simulink model "Quadrotor_PID"  (R2023a)
settings: Solver=VariableStepAuto  StartTime=0.0  StopTime=2000  RelTol=1e-3
model workspace (MAT data in the model file):
  b = 0.000142
  g = 9.8
  m = 1
undefined symbols (not defined in the file or in its folder): Earth, Pitch, Receive, Roll, Send, WGS84, X, Y, Yaw, Z
libraries: slpidlib x6, aerolibfltsims x3, aerolibtransform2 x1
settings Model: Creator=huawei  LastModifiedBy=User
settings SolverCC: ZeroCrossAlgorithm=Adaptive  AlgebraicLoopSolver=TrustRegion
settings DebuggingCC: IgnoredZcDiagnostic=none  UnconnectedInputMsg=warning  UnconnectedOutputMsg=warning  UnconnectedLineMsg=warning
settings ModelReferenceCC: EnableRefExpFcnMdlSchedulingChecks=on
settings RTWCC: DLArmComputeVersion=19.05

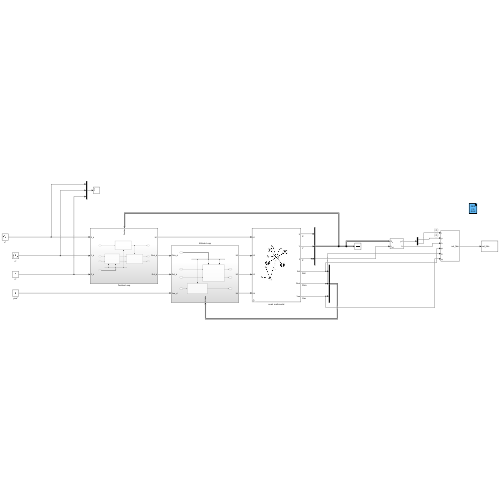
[thumbnail: Simulink's stored preview of the top-level diagram]
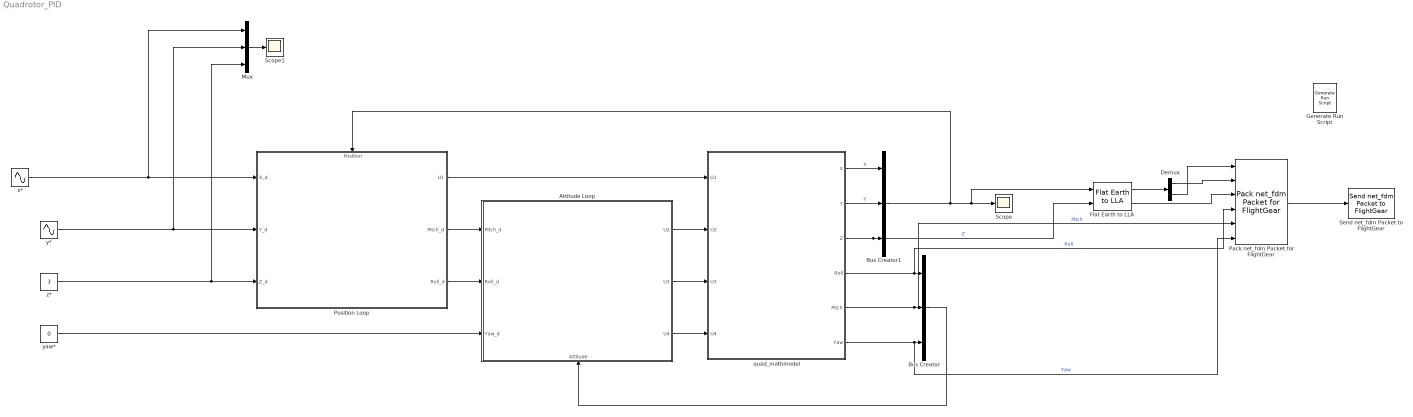
== system Quadrotor_PID ==
  Attitude Loop : Subsystem
      settings: PortSchema="{\"entries\":[{\"content\":{\"sides\":[{\"content\":{\"connectorIds\":[\"In1\",\"In2\",\"In3\"]},\"type\":\"ConnectorPlacement.EquallySpacedRectSide\",\"uuid\":\"741c63cb-3193-49ed-b6fe-0554dd8eb38b\"},{\"content\":{\"connectorIds\":[\"Out1\",\"Out2\",\"Out3\"],\"side\":\"RIGHT\"},\"type\":\"ConnectorPlacement.EquallySpacedRectSide\",\"uuid\":\"55d4e1d6-ced0-4d00-88f3-94ecae3eab08\"},{\"content\":{\"connectorIds\":[],\"side\":\"TOP\"},\"type\":\"ConnectorPlacement.EquallySpacedRectSide\",\"uuid\":\"670d5dfa-1a50-4aee-963c-097076b25aa9\"},{\"content\":{\"connectorIds\":[\"In4\"],\"side\":\"BOTTOM\"},\"type\":\"ConnectorPlacement.EquallySpacedRectSide\",\"uuid\":\"461487f9-9010-46f7-8d40-b6bfcadca1df\"},{\"content\":{\"connectorIds\":[],\"side\":\"HIDDEN\"},\"type\":\"ConnectorPlacement.EquallySpacedRectSide\",\"uuid\":\"46070c40-0b01-41e4-9178-eaa0a7804a93\"}]},\"type\":\"ConnectorPlacement.EquallySpacedConnector\",\"uuid\":\"b0fd4550-2f46-4562-9b6e-a30bcd34312f\"}],\"packageUris\":[\"http://schema.mathworks.com/mf0/Connector/R2020b\"],\"version\":\"1.0\"}"
  Bus Creator : BusCreator  Inputs=Roll,Pitch,Yaw
  Bus Creator1 : BusCreator  Inputs=X,Y,Z
  Demux : Demux  Outputs=2
  Flat Earth to LLA : aerolibtransform2/Flat Earth to LLA  units=Metric (MKS)  ptype=Earth (WGS84)  F=1/298.257223563  R=6378137  refPosPort=off  LL0=[0 10]  psi=0
  Generate Run Script : aerolibfltsims/Generate Run Script  Architecture=Default  dataFlow=Send-Receive  GeometryModelName=c172p  AirportId=KSFO  RunwayId=10L  InitialAltitude=0  InitialHeading=113  OffsetDistance=0  OffsetAzimuth=0  InstallScenery=off  DisableShaders=off  OriginAddress=127.0.0.1  DestinationPort=5502  OriginPort=5505  LocalAddress=127.0.0.1  OutputFileName=runfg.bat  FlightGearBaseDirectory=C:\Program Files\FlightGear 2020.3
  Mux : Mux  Inputs=3
  Pack net_fdm Packet for FlightGear : aerolibfltsims/Pack net_fdm Packet for FlightGear  FlightGearVersion=v2019.1  ShowPositionAttitudeInputs=on  ShowVelocityAccelerationInputs=off  ShowControlSurfacePositionInputs=off  ShowEngineFuelInputs=off  ShowLandingGearInputs=off  ShowEnvironmentInputs=off  SampleTime=-1  packetVersion=24
  Position Loop : Subsystem
      settings: PortSchema="{\"entries\":[{\"content\":{\"sides\":[{\"content\":{\"connectorIds\":[\"In1\",\"In2\",\"In3\"]},\"type\":\"ConnectorPlacement.EquallySpacedRectSide\",\"uuid\":\"741c63cb-3193-49ed-b6fe-0554dd8eb38b\"},{\"content\":{\"connectorIds\":[\"Out1\",\"Out2\",\"Out3\"],\"side\":\"RIGHT\"},\"type\":\"ConnectorPlacement.EquallySpacedRectSide\",\"uuid\":\"55d4e1d6-ced0-4d00-88f3-94ecae3eab08\"},{\"content\":{\"connectorIds\":[\"In4\"],\"side\":\"TOP\"},\"type\":\"ConnectorPlacement.EquallySpacedRectSide\",\"uuid\":\"670d5dfa-1a50-4aee-963c-097076b25aa9\"},{\"content\":{\"connectorIds\":[],\"side\":\"BOTTOM\"},\"type\":\"ConnectorPlacement.EquallySpacedRectSide\",\"uuid\":\"31dc6e32-e4ae-4a63-8318-e80959689dd0\"},{\"content\":{\"connectorIds\":[],\"side\":\"HIDDEN\"},\"type\":\"ConnectorPlacement.EquallySpacedRectSide\",\"uuid\":\"46070c40-0b01-41e4-9178-eaa0a7804a93\"}]},\"type\":\"ConnectorPlacement.EquallySpacedConnector\",\"uuid\":\"b0fd4550-2f46-4562-9b6e-a30bcd34312f\"}],\"packageUris\":[\"http://schema.mathworks.com/mf0/Connector/R2020b\"],\"version\":\"1.0\"}"
  Scope : Scope
  Scope1 : Scope
  Send net_fdm Packet to FlightGear : aerolibfltsims/Send net_fdm Packet to FlightGear  DestinationIpAddress=127.0.0.1  DestinationPort=5502  LocalIpPort=-1  varLen=off  SampleTime=-1
  quad_mathmodel : Subsystem  mask{m=1, L=0.24, b=1.42e-4, d=6.21e-5, g=9.8, Ix=8.1e-3, Iy=8.1e-3, Iz=12.4e-3, Jtp=7.24e-5}
      mask DialogControl ParameterGroupVar Prompt: 四旋翼飞行器参数设置
      mask DialogControl Container10 Prompt: 飞行器质量(kg)
      mask DialogControl Container11 Prompt: 质心到电机中心轴距(m)
      mask DialogControl Container16 Prompt: 升力系数
      mask DialogControl Container15 Prompt: 阻力系数
      mask DialogControl Container14 Prompt: 重力加速度
      mask DialogControl Container13 Prompt: 绕X轴转动惯量
      mask DialogControl Container12 Prompt: 绕Y轴转动惯量
      mask DialogControl Container17 Prompt: 绕Z轴转动惯量
      mask DialogControl Container18 Prompt: 机体绕转轴的总转动惯量（可忽略）
      mask Display: image('$imagefile'); % Use "Edit Image" on toolstrip to change.
  x* : Sin  Frequency=2*pi*.003  Phase=-pi/2  SampleTime=0
  y* : Sin  Frequency=2*pi*.003  SampleTime=0
  yaw* : Constant  Value=0
  z* : Constant  Value=3
  wires:
  quad_mathmodel/3(Z) -> Flat Earth to LLA/2, Bus Creator1/3  "Z"
  Bus Creator1/1 -> Flat Earth to LLA/1, Scope/1, Position Loop/4(Position)
  x*/1 -> Mux/1, Position Loop/1(X_d)
  quad_mathmodel/2(Y) -> Bus Creator1/2  "Y"
  Attitude Loop/3(U4) -> quad_mathmodel/4(U4)
  z*/1 -> Mux/3, Position Loop/3(Z_d)
  Attitude Loop/1(U2) -> quad_mathmodel/2(U2)
  y*/1 -> Mux/2, Position Loop/2(Y_d)
  Position Loop/1(U1) -> quad_mathmodel/1(U1)
  Bus Creator/1 -> Attitude Loop/4(Attitude)
  quad_mathmodel/4(Roll) -> Pack net_fdm Packet for FlightGear/4, Bus Creator/1  "Roll"
  Attitude Loop/2(U3) -> quad_mathmodel/3(U3)
  Position Loop/2(Pitch_d) -> Attitude Loop/1(Pitch_d)
  quad_mathmodel/1(X) -> Bus Creator1/1  "X"
  Position Loop/3(Roll_d) -> Attitude Loop/2(Roll_d)
  quad_mathmodel/5(Pitch) -> Pack net_fdm Packet for FlightGear/5, Bus Creator/2  "Pitch"
  yaw*/1 -> Attitude Loop/3(Yaw_d)
  quad_mathmodel/6(Yaw) -> Pack net_fdm Packet for FlightGear/6, Bus Creator/3  "Yaw"
  Mux/1 -> Scope1/1
  Pack net_fdm Packet for FlightGear/1 -> Send net_fdm Packet to FlightGear/1
  Flat Earth to LLA/1 -> Demux/1
  Demux/1 -> Pack net_fdm Packet for FlightGear/2
  Demux/2 -> Pack net_fdm Packet for FlightGear/1
  Flat Earth to LLA/2 -> Pack net_fdm Packet for FlightGear/3

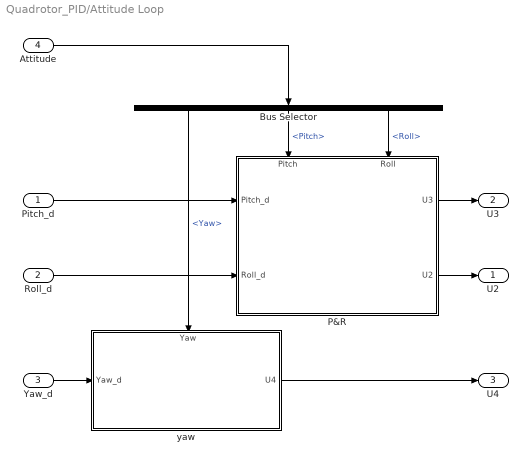
== system Quadrotor_PID/Attitude Loop ==
  Pitch_d : Inport
  Roll_d : Inport  Port=2
  Yaw_d : Inport  Port=3
  Attitude : Inport  Port=4
  Bus Selector : BusSelector  OutputSignals=Yaw,Pitch,Roll
  P&R : Subsystem
      settings: PortSchema="{\"entries\":[{\"content\":{\"sides\":[{\"content\":{\"connectorIds\":[\"In1\",\"In2\"]},\"type\":\"ConnectorPlacement.EquallySpacedRectSide\",\"uuid\":\"5a168f57-9082-4ef9-b723-ec42d235f15b\"},{\"content\":{\"connectorIds\":[\"Out1\",\"Out2\"],\"side\":\"RIGHT\"},\"type\":\"ConnectorPlacement.EquallySpacedRectSide\",\"uuid\":\"1b4dc671-5a32-4537-87d8-64b7817d412d\"},{\"content\":{\"connectorIds\":[\"In3\",\"In4\"],\"side\":\"TOP\"},\"type\":\"ConnectorPlacement.EquallySpacedRectSide\",\"uuid\":\"3d489923-4a97-462b-9fd9-288b2bf2a159\"},{\"content\":{\"connectorIds\":[],\"side\":\"HIDDEN\"},\"type\":\"ConnectorPlacement.EquallySpacedRectSide\",\"uuid\":\"f2e8a974-f6bc-4a20-b9fe-32904cbbc482\"}]},\"type\":\"ConnectorPlacement.EquallySpacedConnector\",\"uuid\":\"91228c47-fce9-4c1d-8a3a-204dc80f90dd\"}],\"packageUris\":[\"http://schema.mathworks.com/mf0/Connector/R2020b\"],\"version\":\"1.0\"}"
  yaw : Subsystem
      settings: PortSchema="{\"entries\":[{\"content\":{\"sides\":[{\"content\":{\"connectorIds\":[\"In1\"]},\"type\":\"ConnectorPlacement.EquallySpacedRectSide\",\"uuid\":\"a7b1533a-1266-40d5-b52c-012082b26468\"},{\"content\":{\"connectorIds\":[\"Out1\"],\"side\":\"RIGHT\"},\"type\":\"ConnectorPlacement.EquallySpacedRectSide\",\"uuid\":\"b4620233-0e85-40ae-9738-c29ba1209ef5\"},{\"content\":{\"connectorIds\":[\"In2\"],\"side\":\"TOP\"},\"type\":\"ConnectorPlacement.EquallySpacedRectSide\",\"uuid\":\"ab9c222c-25de-47f6-b54f-342fd8d0321b\"},{\"content\":{\"connectorIds\":[],\"side\":\"BOTTOM\"},\"type\":\"ConnectorPlacement.EquallySpacedRectSide\",\"uuid\":\"5eacbb93-3d5d-4d57-aaef-fda87c8b1f96\"},{\"content\":{\"connectorIds\":[],\"side\":\"HIDDEN\"},\"type\":\"ConnectorPlacement.EquallySpacedRectSide\",\"uuid\":\"6ed2670f-d779-4b00-b067-d8065a88322b\"}]},\"type\":\"ConnectorPlacement.EquallySpacedConnector\",\"uuid\":\"8cc1c8e9-c992-4e05-8575-ab9d3ec9e6a4\"}],\"packageUris\":[\"http://schema.mathworks.com/mf0/Connector/R2020b\"],\"version\":\"1.0\"}"
  U2 : Outport
  U3 : Outport  Port=2
  U4 : Outport  Port=3
  wires:
  Bus Selector/2 -> P&R/3(Pitch)  "<Pitch>"
  Roll_d/1 -> P&R/2(Roll_d)
  yaw/1(U4) -> U4/1
  Attitude/1 -> Bus Selector/1
  Bus Selector/3 -> P&R/4(Roll)  "<Roll>"
  Pitch_d/1 -> P&R/1(Pitch_d)
  Bus Selector/1 -> yaw/2(Yaw)  "<Yaw>"
  P&R/2(U2) -> U2/1
  P&R/1(U3) -> U3/1
  Yaw_d/1 -> yaw/1(Yaw_d)

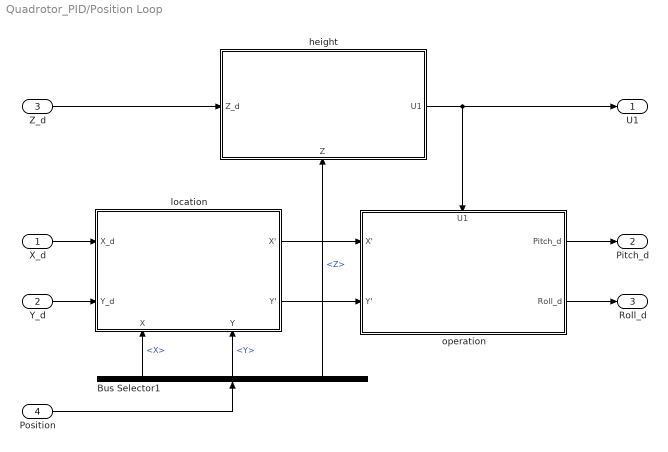
== system Quadrotor_PID/Position Loop ==
  X_d : Inport
  Y_d : Inport  Port=2
  Z_d : Inport  Port=3
  Position : Inport  Port=4
  Bus Selector1 : BusSelector  OutputSignals=X,Y,Z
  height : Subsystem
      settings: PortSchema="{\"entries\":[{\"content\":{\"sides\":[{\"content\":{\"connectorIds\":[\"In1\"]},\"type\":\"ConnectorPlacement.EquallySpacedRectSide\",\"uuid\":\"a7b1533a-1266-40d5-b52c-012082b26468\"},{\"content\":{\"connectorIds\":[\"Out1\"],\"side\":\"RIGHT\"},\"type\":\"ConnectorPlacement.EquallySpacedRectSide\",\"uuid\":\"b4620233-0e85-40ae-9738-c29ba1209ef5\"},{\"content\":{\"connectorIds\":[],\"side\":\"TOP\"},\"type\":\"ConnectorPlacement.EquallySpacedRectSide\",\"uuid\":\"ab9c222c-25de-47f6-b54f-342fd8d0321b\"},{\"content\":{\"connectorIds\":[\"In2\"],\"side\":\"BOTTOM\"},\"type\":\"ConnectorPlacement.EquallySpacedRectSide\",\"uuid\":\"c0ec5864-a2e3-4dc9-86df-2e8e31dc698f\"},{\"content\":{\"connectorIds\":[],\"side\":\"HIDDEN\"},\"type\":\"ConnectorPlacement.EquallySpacedRectSide\",\"uuid\":\"6ed2670f-d779-4b00-b067-d8065a88322b\"}]},\"type\":\"ConnectorPlacement.EquallySpacedConnector\",\"uuid\":\"8cc1c8e9-c992-4e05-8575-ab9d3ec9e6a4\"}],\"packageUris\":[\"http://schema.mathworks.com/mf0/Connector/R2020b\"],\"version\":\"1.0\"}"
  "location " : Subsystem
      settings: PortSchema="{\"entries\":[{\"content\":{\"sides\":[{\"content\":{\"connectorIds\":[\"In1\",\"In2\"]},\"type\":\"ConnectorPlacement.EquallySpacedRectSide\",\"uuid\":\"5a168f57-9082-4ef9-b723-ec42d235f15b\"},{\"content\":{\"connectorIds\":[\"Out1\",\"Out2\"],\"side\":\"RIGHT\"},\"type\":\"ConnectorPlacement.EquallySpacedRectSide\",\"uuid\":\"1b4dc671-5a32-4537-87d8-64b7817d412d\"},{\"content\":{\"connectorIds\":[],\"side\":\"TOP\"},\"type\":\"ConnectorPlacement.EquallySpacedRectSide\",\"uuid\":\"3d489923-4a97-462b-9fd9-288b2bf2a159\"},{\"content\":{\"connectorIds\":[\"In3\",\"In4\"],\"side\":\"BOTTOM\"},\"type\":\"ConnectorPlacement.EquallySpacedRectSide\",\"uuid\":\"ca455ebd-18aa-4cdd-b9a1-332337147b86\"},{\"content\":{\"connectorIds\":[],\"side\":\"HIDDEN\"},\"type\":\"ConnectorPlacement.EquallySpacedRectSide\",\"uuid\":\"f2e8a974-f6bc-4a20-b9fe-32904cbbc482\"}]},\"type\":\"ConnectorPlacement.EquallySpacedConnector\",\"uuid\":\"91228c47-fce9-4c1d-8a3a-204dc80f90dd\"}],\"packageUris\":[\"http://schema.mathworks.com/mf0/Connector/R2020b\"],\"version\":\"1.0\"}"
  operation : Subsystem
      settings: PortSchema="{\"entries\":[{\"content\":{\"sides\":[{\"content\":{\"connectorIds\":[\"In1\",\"In2\"]},\"type\":\"ConnectorPlacement.EquallySpacedRectSide\",\"uuid\":\"7b5ff4eb-d8d0-4c09-9af3-42040e275879\"},{\"content\":{\"connectorIds\":[\"Out1\",\"Out2\"],\"side\":\"RIGHT\"},\"type\":\"ConnectorPlacement.EquallySpacedRectSide\",\"uuid\":\"8346582f-6666-4076-82d0-a237d0151848\"},{\"content\":{\"connectorIds\":[\"In3\"],\"side\":\"TOP\"},\"type\":\"ConnectorPlacement.EquallySpacedRectSide\",\"uuid\":\"392c211c-fa44-4e3a-adf5-1ced3bd87e05\"},{\"content\":{\"connectorIds\":[],\"side\":\"HIDDEN\"},\"type\":\"ConnectorPlacement.EquallySpacedRectSide\",\"uuid\":\"198276da-d589-40b0-b73f-71cfec7294bf\"}]},\"type\":\"ConnectorPlacement.EquallySpacedConnector\",\"uuid\":\"5d751e66-253e-464d-b7a7-9553a5bc15c8\"}],\"packageUris\":[\"http://schema.mathworks.com/mf0/Connector/R2020b\"],\"version\":\"1.0\"}"
  U1 : Outport
  Pitch_d : Outport  Port=2
  Roll_d : Outport  Port=3
  wires:
  "location "/1(X') -> operation/1(X')
  Bus Selector1/3 -> height/2(Z)  "<Z>"
  height/1(U1) -> U1/1, operation/3(U1)
  Bus Selector1/2 -> "location "/4(Y)  "<Y>"
  Z_d/1 -> height/1(Z_d)
  Bus Selector1/1 -> "location "/3(X)  "<X>"
  Position/1 -> Bus Selector1/1
  "location "/2(Y') -> operation/2(Y')
  operation/2(Roll_d) -> Roll_d/1
  X_d/1 -> "location "/1(X_d)
  Y_d/1 -> "location "/2(Y_d)
  operation/1(Pitch_d) -> Pitch_d/1

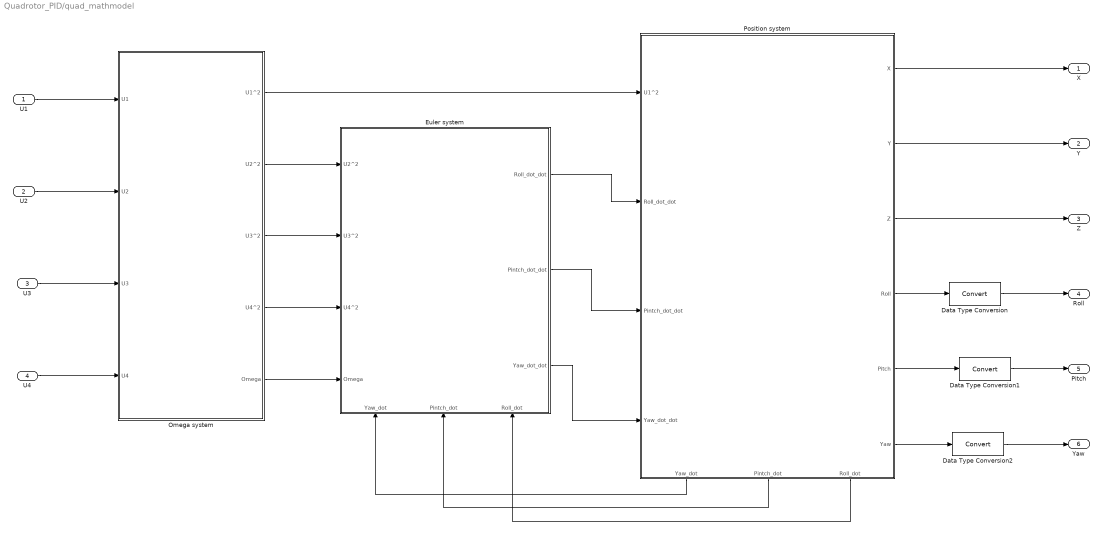
== system Quadrotor_PID/quad_mathmodel ==
  U1 : Inport
  U2 : Inport  Port=2
  U3 : Inport  Port=3
  U4 : Inport  Port=4
  Data Type Conversion : DataTypeConversion  SaturateOnIntegerOverflow=off  RndMeth=Floor
  Data Type Conversion1 : DataTypeConversion  SaturateOnIntegerOverflow=off  RndMeth=Floor
  Data Type Conversion2 : DataTypeConversion  SaturateOnIntegerOverflow=off  RndMeth=Floor
  Euler system : Subsystem
      settings: PortSchema="{\"entries\":[{\"content\":{\"sides\":[{\"content\":{\"connectorIds\":[\"In1\",\"In2\",\"In3\",\"In4\"]},\"type\":\"ConnectorPlacement.EquallySpacedRectSide\",\"uuid\":\"24e9f502-01e2-4796-81d1-4356e5613cd4\"},{\"content\":{\"connectorIds\":[\"Out1\",\"Out2\",\"Out3\"],\"side\":\"RIGHT\"},\"type\":\"ConnectorPlacement.EquallySpacedRectSide\",\"uuid\":\"86fc2a55-a1b7-4625-a7fd-97b1845c6b1e\"},{\"content\":{\"connectorIds\":[],\"side\":\"TOP\"},\"type\":\"ConnectorPlacement.EquallySpacedRectSide\",\"uuid\":\"58e97d03-eced-4c7d-922b-6a4463cc6835\"},{\"content\":{\"connectorIds\":[\"In5\",\"In6\",\"In7\"],\"side\":\"BOTTOM\"},\"type\":\"ConnectorPlacement.EquallySpacedRectSide\",\"uuid\":\"f911275b-2fff-4eb0-817b-81b694121986\"},{\"content\":{\"connectorIds\":[],\"side\":\"HIDDEN\"},\"type\":\"ConnectorPlacement.EquallySpacedRectSide\",\"uuid\":\"f88c6b9c-ef4f-48b0-a4e4-7981c366d7bb\"}]},\"type\":\"ConnectorPlacement.EquallySpacedConnector\",\"uuid\":\"11616862-190a-491d-8e6d-3b18839a1b83\"}],\"packageUris\":[\"http://schema.mathworks.com/mf0/Connector/R2020b\"],\"version\":\"1.0\"}"
  Omega system : Subsystem
  Position system : Subsystem
      settings: PortSchema="{\"entries\":[{\"content\":{\"sides\":[{\"content\":{\"connectorIds\":[\"In1\",\"In2\",\"In3\",\"In4\"]},\"type\":\"ConnectorPlacement.EquallySpacedRectSide\",\"uuid\":\"4e608076-d82c-49dd-b9c3-40de08b530f0\"},{\"content\":{\"connectorIds\":[\"Out1\",\"Out2\",\"Out3\",\"Out4\",\"Out5\",\"Out6\"],\"side\":\"RIGHT\"},\"type\":\"ConnectorPlacement.EquallySpacedRectSide\",\"uuid\":\"79b98a7d-b351-461d-bf57-6a86461ab0e9\"},{\"content\":{\"connectorIds\":[],\"side\":\"TOP\"},\"type\":\"ConnectorPlacement.EquallySpacedRectSide\",\"uuid\":\"a0272396-a878-4308-9d2f-e99a972ffebc\"},{\"content\":{\"connectorIds\":[\"Out7\",\"Out8\",\"Out9\"],\"side\":\"BOTTOM\"},\"type\":\"ConnectorPlacement.EquallySpacedRectSide\",\"uuid\":\"679361ac-afba-4ea2-980e-22b3bd722f7e\"},{\"content\":{\"connectorIds\":[],\"side\":\"HIDDEN\"},\"type\":\"ConnectorPlacement.EquallySpacedRectSide\",\"uuid\":\"68508d46-0468-4fb8-981a-0d305e2aec68\"}]},\"type\":\"ConnectorPlacement.EquallySpacedConnector\",\"uuid\":\"cd6e232c-b153-4628-a51e-54595ea92055\"}],\"packageUris\":[\"http://schema.mathworks.com/mf0/Connector/R2020b\"],\"version\":\"1.0\"}"
  X : Outport
  Y : Outport  Port=2
  Z : Outport  Port=3
  Roll : Outport  Port=4
  Pitch : Outport  Port=5
  Yaw : Outport  Port=6
  wires:
  Position system/6(Yaw) -> Data Type Conversion2/1
  Omega system/5(Omega) -> Euler system/4(Omega)
  Omega system/2(U2^2) -> Euler system/1(U2^2)
  Omega system/3(U3^2) -> Euler system/2(U3^2)
  Position system/2(Y) -> Y/1
  Omega system/1(U1^2) -> Position system/1(U1^2)
  Euler system/2(Pintch_dot_dot) -> Position system/3(Pintch_dot_dot)
  Omega system/4(U4^2) -> Euler system/3(U4^2)
  U3/1 -> Omega system/3(U3)
  Euler system/1(Roll_dot_dot) -> Position system/2(Roll_dot_dot)
  Euler system/3(Yaw_dot_dot) -> Position system/4(Yaw_dot_dot)
  Position system/3(Z) -> Z/1
  U1/1 -> Omega system/1(U1)
  Position system/4(Roll) -> Data Type Conversion/1
  Position system/5(Pitch) -> Data Type Conversion1/1
  Position system/1(X) -> X/1
  U2/1 -> Omega system/2(U2)
  U4/1 -> Omega system/4(U4)
  Position system/9(Roll_dot) -> Euler system/7(Roll_dot)
  Position system/8(Pintch_dot) -> Euler system/6(Pintch_dot)
  Position system/7(Yaw_dot) -> Euler system/5(Yaw_dot)
  Data Type Conversion/1 -> Roll/1
  Data Type Conversion1/1 -> Pitch/1
  Data Type Conversion2/1 -> Yaw/1

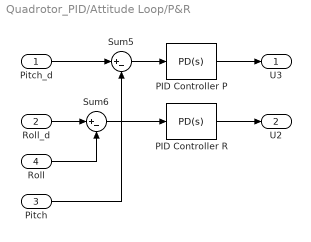
== system Quadrotor_PID/Attitude Loop/P&R ==
  Pitch_d : Inport
  Roll_d : Inport  Port=2
  Pitch : Inport  Port=3
  Roll : Inport  Port=4
  PID Controller P : slpidlib/PID Controller  Controller=PD  Form=Parallel  TimeDomain=Continuous-time  UseExternalTs=off  SampleTime=-1  IntegratorMethod=Forward Euler  FilterMethod=Forward Euler  ControllerParametersSource=internal  P=0.002  I=1.51679966097293e-05  UseKiTs=off  D=0.004  N=3.58143563707461  UseFilter=on  TunerSelectOption=Transfer Function Based (PID Tuner App)  InitialConditionSource=internal  InitialConditionForIntegrator=0  InitialConditionForFilter=0  DifferentiatorICPrevScaledInput=0  ExternalReset=none  TrackingMode=off  Kt=1  LimitOutput=off  SatLimitsSource=internal  UpperSaturationLimit=inf  LowerSaturationLimit=-inf  LinearizeAsGain=on  AntiWindupMode=none  Kb=1  LimitIntegrator=off  UpperIntegratorSaturationLimit=inf  LowerIntegratorSaturationLimit=-inf  POutMin=[]  POutMax=[]  IOutMin=[]  IOutMax=[]  DOutMin=[]  DOutMax=[]  NOutMin=[]  NOutMax=[]  SumOutMin=[]  SumOutMax=[]  SaturationOutMin=[]  SaturationOutMax=[]  PParamMin=[]  PParamMax=[]  IParamMin=[]  IParamMax=[]  DParamMin=[]  DParamMax=[]  NParamMin=[]  NParamMax=[]  KbParamMin=[]  KbParamMax=[]  KtParamMin=[]  KtParamMax=[]  KbOutMin=[]  KbOutMax=[]  KtOutMin=[]  KtOutMax=[]  IntegratorOutMin=[]  IntegratorOutMax=[]  FilterOutMin=[]  FilterOutMax=[]  SumI1OutMin=[]  SumI1OutMax=[]  SumI2OutMin=[]  SumI2OutMax=[]  SumI3OutMin=[]  SumI3OutMax=[]  SumI4OutMin=[]  SumI4OutMax=[]  SumDOutMin=[]  SumDOutMax=[]  DifferentiatorOutMin=[]  DifferentiatorOutMax=[]  FilterDiffOutCoefMin=[]  FilterDiffOutCoefMax=[]  ReciprocalOutMin=[]  ReciprocalOutMax=[]  SumDenOutMin=[]  SumDenOutMax=[]  SumNumOutMin=[]  SumNumOutMax=[]  DivideOutMin=[]  DivideOutMax=[]  UdiffTsProdOutMin=[]  UdiffTsProdOutMax=[]  NTsProdOutMin=[]  NTsProdOutMax=[]  UintegralTsProdOutMin=[]  UintegralTsProdOutMax=[]  UngainTsProdOutMin=[]  UngainTsProdOutMax=[]  ClampingZeroOutDataTypeStr=Inherit: Inherit via back propagation  ClampingZeroOutMin=[]  ClampingZeroOutMax=[]  FilterDenConstantOutDataTypeStr=Inherit: Inherit via back propagation  FilterDenConstantOutMin=[]  FilterDenConstantOutMax=[]  PCopyOutDataTypeStr=Inherit: Inherit via back propagation  PCopyOutMin=[]  PCopyOutMax=[]  NCopyOutDataTypeStr=Inherit: Inherit via back propagation  NCopyOutMin=[]  NCopyOutMax=[]  IntegratorContinuousStateAttributes=''  IntegratorStateMustResolveToSignalObject=off  IntegratorRTWStateStorageClass=Auto  FilterContinuousStateAttributes=''  FilterStateMustResolveToSignalObject=off  FilterRTWStateStorageClass=Auto  ParallelPVariant=InternalParameters  IdealPVariant=Disabled  IVariant=Disabled  DVariant=InternalParameters  IntegratorVariant=Disabled  SatVariant=Disabled  AWVariant=Disabled  PCopyVariant=Disabled  TRVariant=Disabled  FdbkBlocksVariant=Forward  IdealPFdbkVariant=Disabled  SatFdbkVariant=Disabled  DerivativeFilterVariant=ContFilter  NVariant=InternalParameters  NCopyVariant=Disabled  FilterICVariant=InternalICsFilter  IntegratorICVariant=Disabled  ExternalResetVariant=Disabled  TRSumVariant=Passthrough  SumFdbkVariant=Disabled  SumVariant=Sum_PD  TsampFilterVariant=InternalTs  TsampNgainVariant=Passthrough  TsampIntegralVariant=Disabled_SignalSpec  ExternalSaturationOutDataTypeStr=Inherit: Same as second input
  PID Controller R : slpidlib/PID Controller  Controller=PD  Form=Parallel  TimeDomain=Continuous-time  UseExternalTs=off  SampleTime=-1  IntegratorMethod=Forward Euler  FilterMethod=Forward Euler  ControllerParametersSource=internal  P=0.000517944009365722  I=2.09015293720685e-05  UseKiTs=off  D=0.0031516571893313  N=4.69883432592557  UseFilter=on  TunerSelectOption=Transfer Function Based (PID Tuner App)  InitialConditionSource=internal  InitialConditionForIntegrator=0  InitialConditionForFilter=0  DifferentiatorICPrevScaledInput=0  ExternalReset=none  TrackingMode=off  Kt=1  LimitOutput=off  SatLimitsSource=internal  UpperSaturationLimit=inf  LowerSaturationLimit=-inf  LinearizeAsGain=on  AntiWindupMode=none  Kb=1  LimitIntegrator=off  UpperIntegratorSaturationLimit=inf  LowerIntegratorSaturationLimit=-inf  POutMin=[]  POutMax=[]  IOutMin=[]  IOutMax=[]  DOutMin=[]  DOutMax=[]  NOutMin=[]  NOutMax=[]  SumOutMin=[]  SumOutMax=[]  SaturationOutMin=[]  SaturationOutMax=[]  PParamMin=[]  PParamMax=[]  IParamMin=[]  IParamMax=[]  DParamMin=[]  DParamMax=[]  NParamMin=[]  NParamMax=[]  KbParamMin=[]  KbParamMax=[]  KtParamMin=[]  KtParamMax=[]  KbOutMin=[]  KbOutMax=[]  KtOutMin=[]  KtOutMax=[]  IntegratorOutMin=[]  IntegratorOutMax=[]  FilterOutMin=[]  FilterOutMax=[]  SumI1OutMin=[]  SumI1OutMax=[]  SumI2OutMin=[]  SumI2OutMax=[]  SumI3OutMin=[]  SumI3OutMax=[]  SumI4OutMin=[]  SumI4OutMax=[]  SumDOutMin=[]  SumDOutMax=[]  DifferentiatorOutMin=[]  DifferentiatorOutMax=[]  FilterDiffOutCoefMin=[]  FilterDiffOutCoefMax=[]  ReciprocalOutMin=[]  ReciprocalOutMax=[]  SumDenOutMin=[]  SumDenOutMax=[]  SumNumOutMin=[]  SumNumOutMax=[]  DivideOutMin=[]  DivideOutMax=[]  UdiffTsProdOutMin=[]  UdiffTsProdOutMax=[]  NTsProdOutMin=[]  NTsProdOutMax=[]  UintegralTsProdOutMin=[]  UintegralTsProdOutMax=[]  UngainTsProdOutMin=[]  UngainTsProdOutMax=[]  ClampingZeroOutDataTypeStr=Inherit: Inherit via back propagation  ClampingZeroOutMin=[]  ClampingZeroOutMax=[]  FilterDenConstantOutDataTypeStr=Inherit: Inherit via back propagation  FilterDenConstantOutMin=[]  FilterDenConstantOutMax=[]  PCopyOutDataTypeStr=Inherit: Inherit via back propagation  PCopyOutMin=[]  PCopyOutMax=[]  NCopyOutDataTypeStr=Inherit: Inherit via back propagation  NCopyOutMin=[]  NCopyOutMax=[]  IntegratorContinuousStateAttributes=''  IntegratorStateMustResolveToSignalObject=off  IntegratorRTWStateStorageClass=Auto  FilterContinuousStateAttributes=''  FilterStateMustResolveToSignalObject=off  FilterRTWStateStorageClass=Auto  ParallelPVariant=InternalParameters  IdealPVariant=Disabled  IVariant=Disabled  DVariant=InternalParameters  IntegratorVariant=Disabled  SatVariant=Disabled  AWVariant=Disabled  PCopyVariant=Disabled  TRVariant=Disabled  FdbkBlocksVariant=Forward  IdealPFdbkVariant=Disabled  SatFdbkVariant=Disabled  DerivativeFilterVariant=ContFilter  NVariant=InternalParameters  NCopyVariant=Disabled  FilterICVariant=InternalICsFilter  IntegratorICVariant=Disabled  ExternalResetVariant=Disabled  TRSumVariant=Passthrough  SumFdbkVariant=Disabled  SumVariant=Sum_PD  TsampFilterVariant=InternalTs  TsampNgainVariant=Passthrough  TsampIntegralVariant=Disabled_SignalSpec  ExternalSaturationOutDataTypeStr=Inherit: Same as second input
  Sum5 : Sum  Inputs=|+-
  Sum6 : Sum  Inputs=|+-
  U3 : Outport
  U2 : Outport  Port=2
  wires:
  PID Controller P/1 -> U3/1
  Pitch/1 -> Sum5/2
  Sum6/1 -> PID Controller R/1
  Sum5/1 -> PID Controller P/1
  Roll/1 -> Sum6/2
  PID Controller R/1 -> U2/1
  Pitch_d/1 -> Sum5/1
  Roll_d/1 -> Sum6/1

== system Quadrotor_PID/Attitude Loop/yaw ==
  Yaw_d : Inport
  Yaw : Inport  Port=2
  PID Controller Y : slpidlib/PID Controller  Controller=PD  Form=Parallel  TimeDomain=Continuous-time  UseExternalTs=off  SampleTime=-1  IntegratorMethod=Forward Euler  FilterMethod=Forward Euler  ControllerParametersSource=internal  P=0.00070917828540938  I=0  UseKiTs=off  D=0.00337767414842328  N=2.26407668868773  UseFilter=on  TunerSelectOption=Transfer Function Based (PID Tuner App)  InitialConditionSource=internal  InitialConditionForIntegrator=0  InitialConditionForFilter=0  DifferentiatorICPrevScaledInput=0  ExternalReset=none  TrackingMode=off  Kt=1  LimitOutput=off  SatLimitsSource=internal  UpperSaturationLimit=inf  LowerSaturationLimit=-inf  LinearizeAsGain=on  AntiWindupMode=none  Kb=1  LimitIntegrator=off  UpperIntegratorSaturationLimit=inf  LowerIntegratorSaturationLimit=-inf  POutMin=[]  POutMax=[]  IOutMin=[]  IOutMax=[]  DOutMin=[]  DOutMax=[]  NOutMin=[]  NOutMax=[]  SumOutMin=[]  SumOutMax=[]  SaturationOutMin=[]  SaturationOutMax=[]  PParamMin=[]  PParamMax=[]  IParamMin=[]  IParamMax=[]  DParamMin=[]  DParamMax=[]  NParamMin=[]  NParamMax=[]  KbParamMin=[]  KbParamMax=[]  KtParamMin=[]  KtParamMax=[]  KbOutMin=[]  KbOutMax=[]  KtOutMin=[]  KtOutMax=[]  IntegratorOutMin=[]  IntegratorOutMax=[]  FilterOutMin=[]  FilterOutMax=[]  SumI1OutMin=[]  SumI1OutMax=[]  SumI2OutMin=[]  SumI2OutMax=[]  SumI3OutMin=[]  SumI3OutMax=[]  SumI4OutMin=[]  SumI4OutMax=[]  SumDOutMin=[]  SumDOutMax=[]  DifferentiatorOutMin=[]  DifferentiatorOutMax=[]  FilterDiffOutCoefMin=[]  FilterDiffOutCoefMax=[]  ReciprocalOutMin=[]  ReciprocalOutMax=[]  SumDenOutMin=[]  SumDenOutMax=[]  SumNumOutMin=[]  SumNumOutMax=[]  DivideOutMin=[]  DivideOutMax=[]  UdiffTsProdOutMin=[]  UdiffTsProdOutMax=[]  NTsProdOutMin=[]  NTsProdOutMax=[]  UintegralTsProdOutMin=[]  UintegralTsProdOutMax=[]  UngainTsProdOutMin=[]  UngainTsProdOutMax=[]  ClampingZeroOutDataTypeStr=Inherit: Inherit via back propagation  ClampingZeroOutMin=[]  ClampingZeroOutMax=[]  FilterDenConstantOutDataTypeStr=Inherit: Inherit via back propagation  FilterDenConstantOutMin=[]  FilterDenConstantOutMax=[]  PCopyOutDataTypeStr=Inherit: Inherit via back propagation  PCopyOutMin=[]  PCopyOutMax=[]  NCopyOutDataTypeStr=Inherit: Inherit via back propagation  NCopyOutMin=[]  NCopyOutMax=[]  IntegratorContinuousStateAttributes=''  IntegratorStateMustResolveToSignalObject=off  IntegratorRTWStateStorageClass=Auto  FilterContinuousStateAttributes=''  FilterStateMustResolveToSignalObject=off  FilterRTWStateStorageClass=Auto  ParallelPVariant=InternalParameters  IdealPVariant=Disabled  IVariant=Disabled  DVariant=InternalParameters  IntegratorVariant=Disabled  SatVariant=Disabled  AWVariant=Disabled  PCopyVariant=Disabled  TRVariant=Disabled  FdbkBlocksVariant=Forward  IdealPFdbkVariant=Disabled  SatFdbkVariant=Disabled  DerivativeFilterVariant=ContFilter  NVariant=InternalParameters  NCopyVariant=Disabled  FilterICVariant=InternalICsFilter  IntegratorICVariant=Disabled  ExternalResetVariant=Disabled  TRSumVariant=Passthrough  SumFdbkVariant=Disabled  SumVariant=Sum_PD  TsampFilterVariant=InternalTs  TsampNgainVariant=Passthrough  TsampIntegralVariant=Disabled_SignalSpec  ExternalSaturationOutDataTypeStr=Inherit: Same as second input
  Sum2 : Sum  Inputs=|+-
  U4 : Outport
  wires:
  Yaw/1 -> Sum2/2
  Sum2/1 -> PID Controller Y/1
  Yaw_d/1 -> Sum2/1
  PID Controller Y/1 -> U4/1

== system Quadrotor_PID/Position Loop/height ==
  Z_d : Inport
  Z : Inport  Port=2
  Constant : Constant  Value=g
  PID Controller Z : slpidlib/PID Controller  Controller=PID  Form=Parallel  TimeDomain=Continuous-time  UseExternalTs=off  SampleTime=-1  IntegratorMethod=Forward Euler  FilterMethod=Forward Euler  ControllerParametersSource=internal  P=3.53804542303513  I=0.723013447865675  UseKiTs=off  D=4.25131927818495  N=23.8074436453229  UseFilter=on  TunerSelectOption=Transfer Function Based (PID Tuner App)  InitialConditionSource=internal  InitialConditionForIntegrator=0  InitialConditionForFilter=0  DifferentiatorICPrevScaledInput=0  ExternalReset=none  TrackingMode=off  Kt=1  LimitOutput=off  SatLimitsSource=internal  UpperSaturationLimit=inf  LowerSaturationLimit=-inf  LinearizeAsGain=on  AntiWindupMode=none  Kb=1  LimitIntegrator=off  UpperIntegratorSaturationLimit=inf  LowerIntegratorSaturationLimit=-inf  POutMin=[]  POutMax=[]  IOutMin=[]  IOutMax=[]  DOutMin=[]  DOutMax=[]  NOutMin=[]  NOutMax=[]  SumOutMin=[]  SumOutMax=[]  SaturationOutMin=[]  SaturationOutMax=[]  PParamMin=[]  PParamMax=[]  IParamMin=[]  IParamMax=[]  DParamMin=[]  DParamMax=[]  NParamMin=[]  NParamMax=[]  KbParamMin=[]  KbParamMax=[]  KtParamMin=[]  KtParamMax=[]  KbOutMin=[]  KbOutMax=[]  KtOutMin=[]  KtOutMax=[]  IntegratorOutMin=[]  IntegratorOutMax=[]  FilterOutMin=[]  FilterOutMax=[]  SumI1OutMin=[]  SumI1OutMax=[]  SumI2OutMin=[]  SumI2OutMax=[]  SumI3OutMin=[]  SumI3OutMax=[]  SumI4OutMin=[]  SumI4OutMax=[]  SumDOutMin=[]  SumDOutMax=[]  DifferentiatorOutMin=[]  DifferentiatorOutMax=[]  FilterDiffOutCoefMin=[]  FilterDiffOutCoefMax=[]  ReciprocalOutMin=[]  ReciprocalOutMax=[]  SumDenOutMin=[]  SumDenOutMax=[]  SumNumOutMin=[]  SumNumOutMax=[]  DivideOutMin=[]  DivideOutMax=[]  UdiffTsProdOutMin=[]  UdiffTsProdOutMax=[]  NTsProdOutMin=[]  NTsProdOutMax=[]  UintegralTsProdOutMin=[]  UintegralTsProdOutMax=[]  UngainTsProdOutMin=[]  UngainTsProdOutMax=[]  ClampingZeroOutDataTypeStr=Inherit: Inherit via back propagation  ClampingZeroOutMin=[]  ClampingZeroOutMax=[]  FilterDenConstantOutDataTypeStr=Inherit: Inherit via back propagation  FilterDenConstantOutMin=[]  FilterDenConstantOutMax=[]  PCopyOutDataTypeStr=Inherit: Inherit via back propagation  PCopyOutMin=[]  PCopyOutMax=[]  NCopyOutDataTypeStr=Inherit: Inherit via back propagation  NCopyOutMin=[]  NCopyOutMax=[]  IntegratorContinuousStateAttributes=''  IntegratorStateMustResolveToSignalObject=off  IntegratorRTWStateStorageClass=Auto  FilterContinuousStateAttributes=''  FilterStateMustResolveToSignalObject=off  FilterRTWStateStorageClass=Auto  ParallelPVariant=InternalParameters  IdealPVariant=Disabled  IVariant=InternalParameters  DVariant=InternalParameters  IntegratorVariant=Continuous  SatVariant=Disabled  AWVariant=Passthrough  PCopyVariant=Disabled  TRVariant=Disabled  FdbkBlocksVariant=Forward  IdealPFdbkVariant=Disabled  SatFdbkVariant=Disabled  DerivativeFilterVariant=ContFilter  NVariant=InternalParameters  NCopyVariant=Disabled  FilterICVariant=InternalICsFilter  IntegratorICVariant=InternalICs  ExternalResetVariant=Disabled  TRSumVariant=Passthrough  SumFdbkVariant=Disabled  SumVariant=Sum_PID  TsampFilterVariant=InternalTs  TsampNgainVariant=Passthrough  TsampIntegralVariant=Disabled_SignalSpec  ExternalSaturationOutDataTypeStr=Inherit: Same as second input
  Sum : Sum  Inputs=-+|
  Sum1 : Sum  Inputs=++|
  U1 : Outport
  wires:
  Z/1 -> Sum/1
  Z_d/1 -> Sum/2
  Constant/1 -> Sum1/1
  Sum/1 -> PID Controller Z/1
  PID Controller Z/1 -> Sum1/2
  Sum1/1 -> U1/1

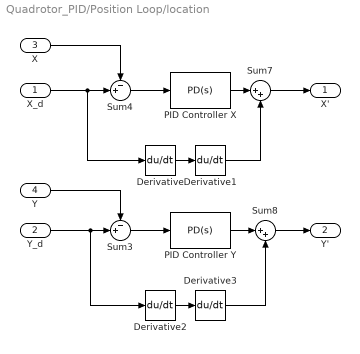
== system Quadrotor_PID/Position Loop/location  ==
  X_d : Inport
  Y_d : Inport  Port=2
  X : Inport  Port=3
  Y : Inport  Port=4
  Derivative{,1..3} (4 alike) : Derivative
  PID Controller X : slpidlib/PID Controller  Controller=PD  Form=Parallel  TimeDomain=Continuous-time  UseExternalTs=off  SampleTime=-1  IntegratorMethod=Forward Euler  FilterMethod=Forward Euler  ControllerParametersSource=internal  P=0.0025  I=1.32852953365654e-05  UseKiTs=off  D=0.13  N=0.173869187987419  UseFilter=on  TunerSelectOption=Transfer Function Based (PID Tuner App)  InitialConditionSource=internal  InitialConditionForIntegrator=0  InitialConditionForFilter=0  DifferentiatorICPrevScaledInput=0  ExternalReset=none  TrackingMode=off  Kt=1  LimitOutput=off  SatLimitsSource=internal  UpperSaturationLimit=inf  LowerSaturationLimit=-inf  LinearizeAsGain=on  AntiWindupMode=none  Kb=1  LimitIntegrator=off  UpperIntegratorSaturationLimit=inf  LowerIntegratorSaturationLimit=-inf  POutMin=[]  POutMax=[]  IOutMin=[]  IOutMax=[]  DOutMin=[]  DOutMax=[]  NOutMin=[]  NOutMax=[]  SumOutMin=[]  SumOutMax=[]  SaturationOutMin=[]  SaturationOutMax=[]  PParamMin=[]  PParamMax=[]  IParamMin=[]  IParamMax=[]  DParamMin=[]  DParamMax=[]  NParamMin=[]  NParamMax=[]  KbParamMin=[]  KbParamMax=[]  KtParamMin=[]  KtParamMax=[]  KbOutMin=[]  KbOutMax=[]  KtOutMin=[]  KtOutMax=[]  IntegratorOutMin=[]  IntegratorOutMax=[]  FilterOutMin=[]  FilterOutMax=[]  SumI1OutMin=[]  SumI1OutMax=[]  SumI2OutMin=[]  SumI2OutMax=[]  SumI3OutMin=[]  SumI3OutMax=[]  SumI4OutMin=[]  SumI4OutMax=[]  SumDOutMin=[]  SumDOutMax=[]  DifferentiatorOutMin=[]  DifferentiatorOutMax=[]  FilterDiffOutCoefMin=[]  FilterDiffOutCoefMax=[]  ReciprocalOutMin=[]  ReciprocalOutMax=[]  SumDenOutMin=[]  SumDenOutMax=[]  SumNumOutMin=[]  SumNumOutMax=[]  DivideOutMin=[]  DivideOutMax=[]  UdiffTsProdOutMin=[]  UdiffTsProdOutMax=[]  NTsProdOutMin=[]  NTsProdOutMax=[]  UintegralTsProdOutMin=[]  UintegralTsProdOutMax=[]  UngainTsProdOutMin=[]  UngainTsProdOutMax=[]  ClampingZeroOutDataTypeStr=Inherit: Inherit via back propagation  ClampingZeroOutMin=[]  ClampingZeroOutMax=[]  FilterDenConstantOutDataTypeStr=Inherit: Inherit via back propagation  FilterDenConstantOutMin=[]  FilterDenConstantOutMax=[]  PCopyOutDataTypeStr=Inherit: Inherit via back propagation  PCopyOutMin=[]  PCopyOutMax=[]  NCopyOutDataTypeStr=Inherit: Inherit via back propagation  NCopyOutMin=[]  NCopyOutMax=[]  IntegratorContinuousStateAttributes=''  IntegratorStateMustResolveToSignalObject=off  IntegratorRTWStateStorageClass=Auto  FilterContinuousStateAttributes=''  FilterStateMustResolveToSignalObject=off  FilterRTWStateStorageClass=Auto  ParallelPVariant=InternalParameters  IdealPVariant=Disabled  IVariant=Disabled  DVariant=InternalParameters  IntegratorVariant=Disabled  SatVariant=Disabled  AWVariant=Disabled  PCopyVariant=Disabled  TRVariant=Disabled  FdbkBlocksVariant=Forward  IdealPFdbkVariant=Disabled  SatFdbkVariant=Disabled  DerivativeFilterVariant=ContFilter  NVariant=InternalParameters  NCopyVariant=Disabled  FilterICVariant=InternalICsFilter  IntegratorICVariant=Disabled  ExternalResetVariant=Disabled  TRSumVariant=Passthrough  SumFdbkVariant=Disabled  SumVariant=Sum_PD  TsampFilterVariant=InternalTs  TsampNgainVariant=Passthrough  TsampIntegralVariant=Disabled_SignalSpec  ExternalSaturationOutDataTypeStr=Inherit: Same as second input
  PID Controller Y : slpidlib/PID Controller  Controller=PD  Form=Parallel  TimeDomain=Continuous-time  UseExternalTs=off  SampleTime=-1  IntegratorMethod=Forward Euler  FilterMethod=Forward Euler  ControllerParametersSource=internal  P=0.01  I=2.10922571180575e-05  UseKiTs=off  D=0.16  N=9.20175473255031  UseFilter=on  TunerSelectOption=Transfer Function Based (PID Tuner App)  InitialConditionSource=internal  InitialConditionForIntegrator=0  InitialConditionForFilter=0  DifferentiatorICPrevScaledInput=0  ExternalReset=none  TrackingMode=off  Kt=1  LimitOutput=off  SatLimitsSource=internal  UpperSaturationLimit=inf  LowerSaturationLimit=-inf  LinearizeAsGain=on  AntiWindupMode=none  Kb=1  LimitIntegrator=off  UpperIntegratorSaturationLimit=inf  LowerIntegratorSaturationLimit=-inf  POutMin=[]  POutMax=[]  IOutMin=[]  IOutMax=[]  DOutMin=[]  DOutMax=[]  NOutMin=[]  NOutMax=[]  SumOutMin=[]  SumOutMax=[]  SaturationOutMin=[]  SaturationOutMax=[]  PParamMin=[]  PParamMax=[]  IParamMin=[]  IParamMax=[]  DParamMin=[]  DParamMax=[]  NParamMin=[]  NParamMax=[]  KbParamMin=[]  KbParamMax=[]  KtParamMin=[]  KtParamMax=[]  KbOutMin=[]  KbOutMax=[]  KtOutMin=[]  KtOutMax=[]  IntegratorOutMin=[]  IntegratorOutMax=[]  FilterOutMin=[]  FilterOutMax=[]  SumI1OutMin=[]  SumI1OutMax=[]  SumI2OutMin=[]  SumI2OutMax=[]  SumI3OutMin=[]  SumI3OutMax=[]  SumI4OutMin=[]  SumI4OutMax=[]  SumDOutMin=[]  SumDOutMax=[]  DifferentiatorOutMin=[]  DifferentiatorOutMax=[]  FilterDiffOutCoefMin=[]  FilterDiffOutCoefMax=[]  ReciprocalOutMin=[]  ReciprocalOutMax=[]  SumDenOutMin=[]  SumDenOutMax=[]  SumNumOutMin=[]  SumNumOutMax=[]  DivideOutMin=[]  DivideOutMax=[]  UdiffTsProdOutMin=[]  UdiffTsProdOutMax=[]  NTsProdOutMin=[]  NTsProdOutMax=[]  UintegralTsProdOutMin=[]  UintegralTsProdOutMax=[]  UngainTsProdOutMin=[]  UngainTsProdOutMax=[]  ClampingZeroOutDataTypeStr=Inherit: Inherit via back propagation  ClampingZeroOutMin=[]  ClampingZeroOutMax=[]  FilterDenConstantOutDataTypeStr=Inherit: Inherit via back propagation  FilterDenConstantOutMin=[]  FilterDenConstantOutMax=[]  PCopyOutDataTypeStr=Inherit: Inherit via back propagation  PCopyOutMin=[]  PCopyOutMax=[]  NCopyOutDataTypeStr=Inherit: Inherit via back propagation  NCopyOutMin=[]  NCopyOutMax=[]  IntegratorContinuousStateAttributes=''  IntegratorStateMustResolveToSignalObject=off  IntegratorRTWStateStorageClass=Auto  FilterContinuousStateAttributes=''  FilterStateMustResolveToSignalObject=off  FilterRTWStateStorageClass=Auto  ParallelPVariant=InternalParameters  IdealPVariant=Disabled  IVariant=Disabled  DVariant=InternalParameters  IntegratorVariant=Disabled  SatVariant=Disabled  AWVariant=Disabled  PCopyVariant=Disabled  TRVariant=Disabled  FdbkBlocksVariant=Forward  IdealPFdbkVariant=Disabled  SatFdbkVariant=Disabled  DerivativeFilterVariant=ContFilter  NVariant=InternalParameters  NCopyVariant=Disabled  FilterICVariant=InternalICsFilter  IntegratorICVariant=Disabled  ExternalResetVariant=Disabled  TRSumVariant=Passthrough  SumFdbkVariant=Disabled  SumVariant=Sum_PD  TsampFilterVariant=InternalTs  TsampNgainVariant=Passthrough  TsampIntegralVariant=Disabled_SignalSpec  ExternalSaturationOutDataTypeStr=Inherit: Same as second input
  Sum3 : Sum  Inputs=-+|
  Sum4 : Sum  Inputs=-+|
  Sum7 : Sum  Inputs=|++
  Sum8 : Sum  Inputs=|++
  X' : Outport
  Y' : Outport  Port=2
  wires:
  Derivative2/1 -> Derivative3/1
  Sum8/1 -> Y'/1
  Derivative1/1 -> Sum7/2
  Derivative/1 -> Derivative1/1
  Derivative3/1 -> Sum8/2
  X_d/1 -> Sum4/2, Derivative/1
  Y_d/1 -> Sum3/2, Derivative2/1
  Sum4/1 -> PID Controller X/1
  PID Controller Y/1 -> Sum8/1
  Sum3/1 -> PID Controller Y/1
  PID Controller X/1 -> Sum7/1
  Sum7/1 -> X'/1
  X/1 -> Sum4/1
  Y/1 -> Sum3/1

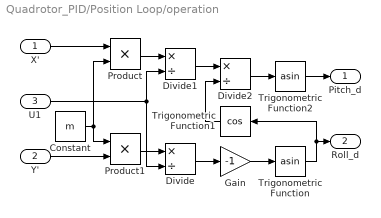
== system Quadrotor_PID/Position Loop/operation ==
  X' : Inport
  Y' : Inport  Port=2
  U1 : Inport  Port=3
  Constant : Constant  Value=m
  Divide : Product  Inputs=*/
  Divide1 : Product  Inputs=*/
  Divide2 : Product  Inputs=*/
  Gain : Gain  Gain=-1
  Product : Product
  Product1 : Product
  Trigonometric Function : Trigonometry  Operator=asin
  Trigonometric Function1 : Trigonometry  Operator=cos
  Trigonometric Function2 : Trigonometry  Operator=asin
  Pitch_d : Outport
  Roll_d : Outport  Port=2
  wires:
  Divide2/1 -> Trigonometric Function2/1
  U1/1 -> Divide1/2, Divide/2
  Divide/1 -> Gain/1
  Trigonometric Function/1 -> Roll_d/1, Trigonometric Function1/1
  Gain/1 -> Trigonometric Function/1
  Trigonometric Function2/1 -> Pitch_d/1
  Trigonometric Function1/1 -> Divide2/2
  Divide1/1 -> Divide2/1
  Product/1 -> Divide1/1
  Product1/1 -> Divide/1
  X'/1 -> Product/1
  Y'/1 -> Product1/2
  Constant/1 -> Product/2, Product1/1

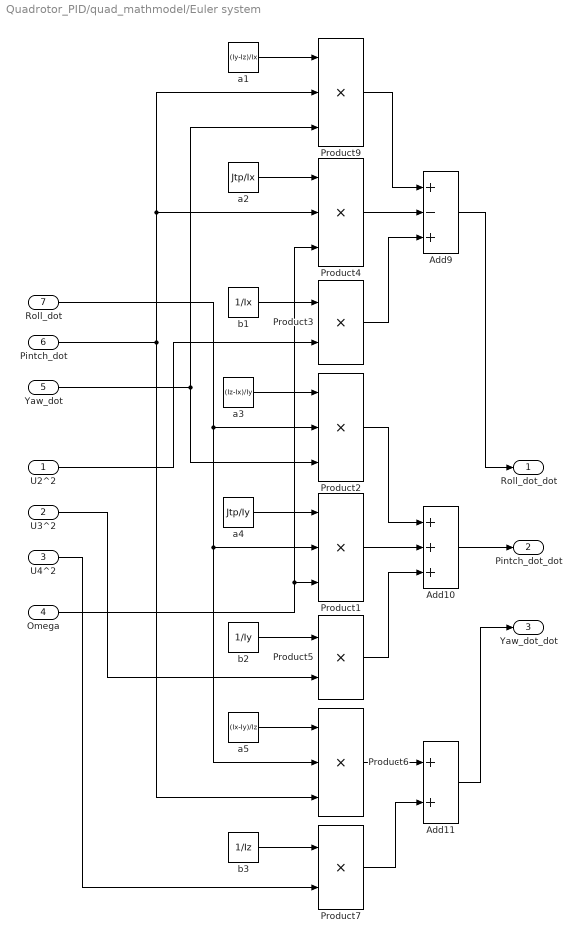
== system Quadrotor_PID/quad_mathmodel/Euler system ==
  U2^2 : Inport
  U3^2 : Inport  Port=2
  U4^2 : Inport  Port=3
  Omega : Inport  Port=4
  Yaw_dot : Inport  Port=5
  Pintch_dot : Inport  Port=6
  Roll_dot : Inport  Port=7
  Add10 : Sum  Inputs=+++
  Add11 : Sum
  Add9 : Sum  Inputs=+-+
  Product{1..2,4,6,9} (5 alike) : Product  Inputs=3
  Product3 : Product
  Product5 : Product
  Product7 : Product
  a1 : Constant  Value=(Iy-Iz)/Ix
  a2 : Constant  Value=Jtp/Ix
  a3 : Constant  Value=(Iz-Ix)/Iy
  a4 : Constant  Value=Jtp/Iy
  a5 : Constant  Value=(Ix-Iy)/Iz
  b1 : Constant  Value=1/Ix
  b2 : Constant  Value=1/Iy
  b3 : Constant  Value=1/Iz
  Roll_dot_dot : Outport
  Pintch_dot_dot : Outport  Port=2
  Yaw_dot_dot : Outport  Port=3
  wires:
  U2^2/1 -> Product3/2
  Product7/1 -> Add11/2
  Product6/1 -> Add11/1
  Product4/1 -> Add9/2
  Product5/1 -> Add10/3
  a1/1 -> Product9/1
  Add10/1 -> Pintch_dot_dot/1
  a2/1 -> Product4/1
  Pintch_dot/1 -> Product6/3, Product9/2, Product4/2
  Yaw_dot/1 -> Product2/3, Product9/3
  Add11/1 -> Yaw_dot_dot/1
  Product2/1 -> Add10/1
  Omega/1 -> Product4/3, Product1/3
  a5/1 -> Product6/1
  b3/1 -> Product7/1
  a4/1 -> Product1/1
  Roll_dot/1 -> Product2/2, Product1/2, Product6/2
  Product1/1 -> Add10/2
  a3/1 -> Product2/1
  b1/1 -> Product3/1
  Product3/1 -> Add9/3
  b2/1 -> Product5/1
  Product9/1 -> Add9/1
  Add9/1 -> Roll_dot_dot/1
  U3^2/1 -> Product5/2
  U4^2/1 -> Product7/2

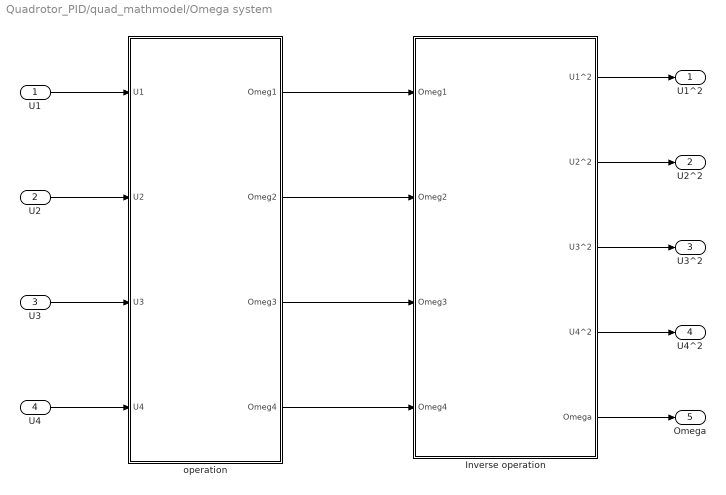
== system Quadrotor_PID/quad_mathmodel/Omega system ==
  U1 : Inport
  U2 : Inport  Port=2
  U3 : Inport  Port=3
  U4 : Inport  Port=4
  Inverse operation : Subsystem
  operation : Subsystem
  U1^2 : Outport
  U2^2 : Outport  Port=2
  U3^2 : Outport  Port=3
  U4^2 : Outport  Port=4
  Omega : Outport  Port=5
  wires:
  Inverse operation/1(U1^2) -> U1^2/1
  Inverse operation/2(U2^2) -> U2^2/1
  Inverse operation/3(U3^2) -> U3^2/1
  Inverse operation/4(U4^2) -> U4^2/1
  Inverse operation/5(Omega) -> Omega/1
  U1/1 -> operation/1(U1)
  U2/1 -> operation/2(U2)
  U3/1 -> operation/3(U3)
  U4/1 -> operation/4(U4)
  operation/1(Omeg1) -> Inverse operation/1(Omeg1)
  operation/2(Omeg2) -> Inverse operation/2(Omeg2)
  operation/3(Omeg3) -> Inverse operation/3(Omeg3)
  operation/4(Omeg4) -> Inverse operation/4(Omeg4)

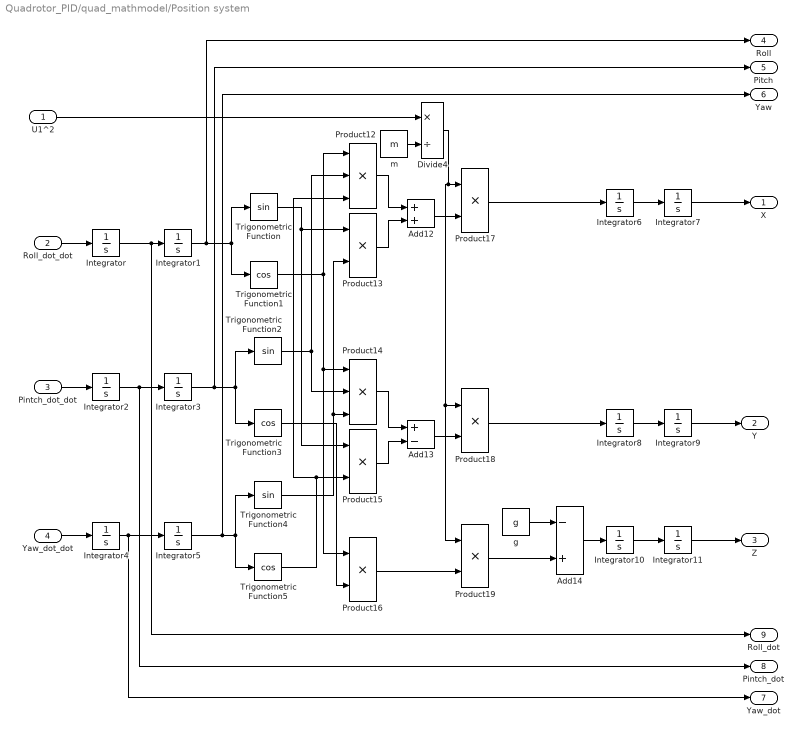
== system Quadrotor_PID/quad_mathmodel/Position system ==
  U1^2 : Inport
  Roll_dot_dot : Inport  Port=2
  Pintch_dot_dot : Inport  Port=3
  Yaw_dot_dot : Inport  Port=4
  Add12 : Sum
  Add13 : Sum  Inputs=+-
  Add14 : Sum  Inputs=-+
  Divide4 : Product  Inputs=*/
  Integrator{,1..11} (12 alike) : Integrator
  Product12 : Product  Inputs=3
  Product{13,15..19} (6 alike) : Product
  Product14 : Product  Inputs=3
  Trigonometric Function : Trigonometry
  Trigonometric Function1 : Trigonometry  Operator=cos
  Trigonometric Function2 : Trigonometry
  Trigonometric Function3 : Trigonometry  Operator=cos
  Trigonometric Function4 : Trigonometry
  Trigonometric Function5 : Trigonometry  Operator=cos
  g : Constant  Value=g
  m : Constant  Value=m
  X : Outport
  Y : Outport  Port=2
  Z : Outport  Port=3
  Roll : Outport  Port=4
  Pitch : Outport  Port=5
  Yaw : Outport  Port=6
  Yaw_dot : Outport  Port=7
  Pintch_dot : Outport  Port=8
  Roll_dot : Outport  Port=9
  wires:
  Integrator10/1 -> Integrator11/1
  Integrator1/1 -> Roll/1, Trigonometric Function1/1, Trigonometric Function/1
  Trigonometric Function/1 -> Product15/1, Product13/1
  Integrator2/1 -> Pintch_dot/1, Integrator3/1
  Integrator3/1 -> Pitch/1, Trigonometric Function2/1, Trigonometric Function3/1
  Add14/1 -> Integrator10/1
  m/1 -> Divide4/2
  Trigonometric Function1/1 -> Product16/1, Product14/1, Product12/1
  Product19/1 -> Add14/2
  Product15/1 -> Add13/2
  Integrator5/1 -> Yaw/1, Trigonometric Function5/1, Trigonometric Function4/1
  Integrator/1 -> Roll_dot/1, Integrator1/1
  Product16/1 -> Product19/2
  Trigonometric Function2/1 -> Product14/2, Product12/2
  Product14/1 -> Add13/1
  Product13/1 -> Add12/2
  Integrator4/1 -> Yaw_dot/1, Integrator5/1
  Pintch_dot_dot/1 -> Integrator2/1
  Trigonometric Function4/1 -> Product13/2, Product14/3
  g/1 -> Add14/1
  Trigonometric Function5/1 -> Product12/3, Product15/2
  Add12/1 -> Product17/2
  Integrator7/1 -> X/1
  Product12/1 -> Add12/1
  Product18/1 -> Integrator8/1
  Product17/1 -> Integrator6/1
  Add13/1 -> Product18/2
  Roll_dot_dot/1 -> Integrator/1
  Divide4/1 -> Product19/1, Product18/1, Product17/1
  Integrator6/1 -> Integrator7/1
  Integrator8/1 -> Integrator9/1
  Trigonometric Function3/1 -> Product16/2
  Yaw_dot_dot/1 -> Integrator4/1
  U1^2/1 -> Divide4/1
  Integrator9/1 -> Y/1
  Integrator11/1 -> Z/1

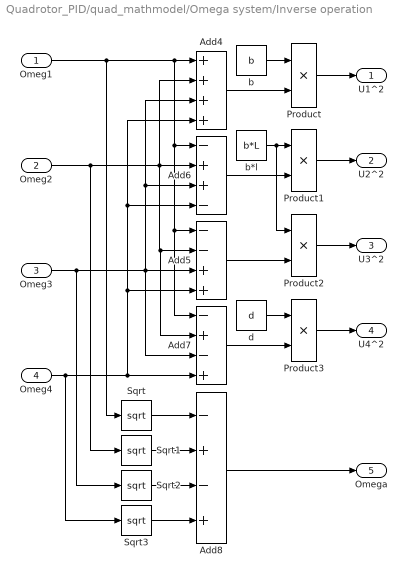
== system Quadrotor_PID/quad_mathmodel/Omega system/Inverse operation ==
  Omeg1 : Inport
  Omeg2 : Inport  Port=2
  Omeg3 : Inport  Port=3
  Omeg4 : Inport  Port=4
  Add4 : Sum  Inputs=++++
  Add5 : Sum  Inputs=--++
  Add6 : Sum  Inputs=-++-
  Add7 : Sum  Inputs=-+-+
  Add8 : Sum  Inputs=-+-+
  Product{,1..3} (4 alike) : Product
  Sqrt{,1..3} (4 alike) : Sqrt
  b : Constant  Value=b
  b*l : Constant  Value=b*L
  d : Constant  Value=d
  U1^2 : Outport
  U2^2 : Outport  Port=2
  U3^2 : Outport  Port=3
  U4^2 : Outport  Port=4
  Omega : Outport  Port=5
  wires:
  Omeg1/1 -> Add7/1, Add5/1, Add6/1, Add4/1, Sqrt/1
  Product2/1 -> U3^2/1
  Add5/1 -> Product2/2
  Add8/1 -> Omega/1
  Product3/1 -> U4^2/1
  Add6/1 -> Product1/2
  b/1 -> Product/1
  Add4/1 -> Product/2
  Omeg4/1 -> Sqrt3/1, Add5/4, Add6/4, Add4/4, Add7/4
  b*l/1 -> Product2/1, Product1/1
  Product1/1 -> U2^2/1
  d/1 -> Product3/1
  Sqrt/1 -> Add8/1
  Sqrt3/1 -> Add8/4
  Omeg3/1 -> Sqrt2/1, Add7/3, Add6/3, Add4/3, Add5/3
  Omeg2/1 -> Sqrt1/1, Add7/2, Add5/2, Add4/2, Add6/2
  Sqrt1/1 -> Add8/2
  Add7/1 -> Product3/2
  Sqrt2/1 -> Add8/3
  Product/1 -> U1^2/1

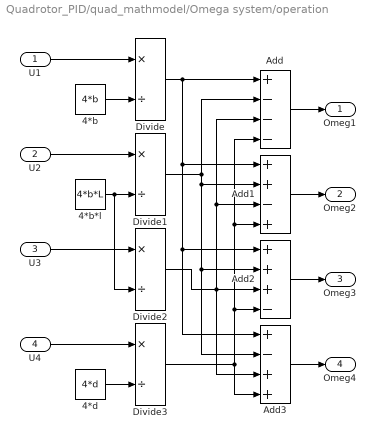
== system Quadrotor_PID/quad_mathmodel/Omega system/operation ==
  U1 : Inport
  U2 : Inport  Port=2
  U3 : Inport  Port=3
  U4 : Inport  Port=4
  4*b : Constant  Value=4*b
  4*b*l : Constant  Value=4*b*L
  4*d : Constant  Value=4*d
  Add : Sum  Inputs=+---
  Add1 : Sum  Inputs=++-+
  Add2 : Sum  Inputs=+++-
  Add3 : Sum  Inputs=+-++
  Divide{,1..3} (4 alike) : Product  Inputs=*/
  Omeg1 : Outport
  Omeg2 : Outport  Port=2
  Omeg3 : Outport  Port=3
  Omeg4 : Outport  Port=4
  wires:
  U1/1 -> Divide/1
  4*b*l/1 -> Divide2/2, Divide1/2
  U3/1 -> Divide2/1
  Divide3/1 -> Add3/4, Add/4, Add1/4, Add2/4
  U2/1 -> Divide1/1
  Divide1/1 -> Add3/2, Add2/2, Add1/2, Add/2
  Add1/1 -> Omeg2/1
  4*d/1 -> Divide3/2
  Divide2/1 -> Add2/3, Add3/3, Add1/3, Add/3
  Divide/1 -> Add/1, Add1/1, Add2/1, Add3/1
  4*b/1 -> Divide/2
  U4/1 -> Divide3/1
  Add3/1 -> Omeg4/1
  Add2/1 -> Omeg3/1
  Add/1 -> Omeg1/1
